simulink model "HinfModelLinear"  (R2018b)
settings: Solver=VariableStepAuto  StartTime=0.0  StopTime=20  RelTol=1e-3
undefined symbols (not defined in the file): A, B1, B2, C, K
libraries: cstblocks x1
settings Model: Creator=jban039  LastModifiedBy=jban039

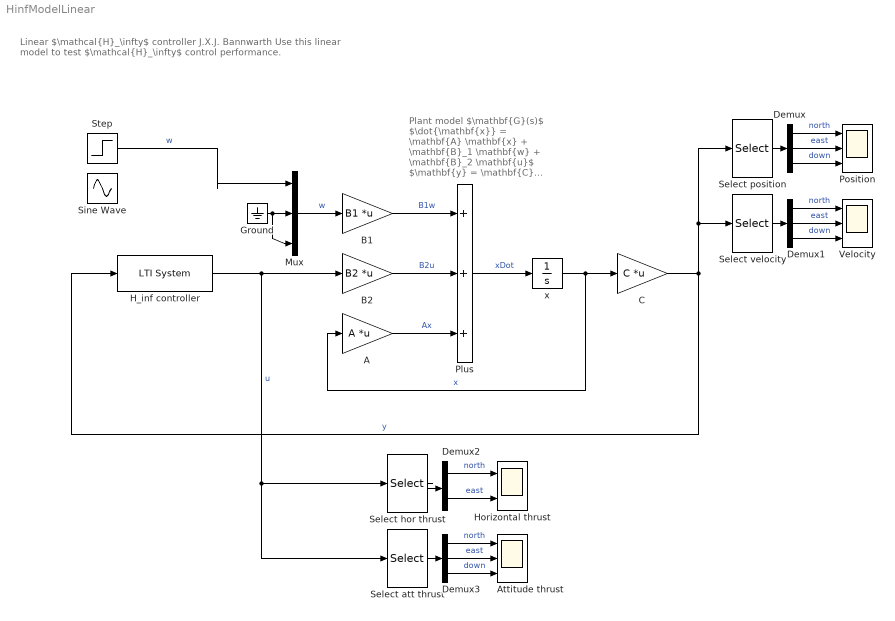
== system HinfModelLinear ==
  note: Linear $\mathcal{H}_\infty$ controller
      | J.X.J. Bannwarth
      |
      | Use this linear model to test $\mathcal{H}_\infty$ control performance.
  note: Plant model
      | $\mathbf{G}(s)$
      | $\dot{\mathbf{x}} = \mathbf{A} \mathbf{x} + \mathbf{B}_1 \mathbf{w} + \mathbf{B}_2 \mathbf{u}$
      | $\mathbf{y} = \mathbf{C} \mathbf{x}$
  A : Gain  Gain=A  Multiplication=Matrix(K*u)
  Attitude thrust : Scope  NumInputPorts=3
  B1 : Gain  Gain=B1  Multiplication=Matrix(K*u)
  B2 : Gain  Gain=B2  Multiplication=Matrix(K*u)
  C : Gain  Gain=C  Multiplication=Matrix(K*u)
  Demux : Demux  Outputs=3
  Demux1 : Demux  Outputs=3
  Demux2 : Demux  Outputs=2
  Demux3 : Demux  Outputs=3
  Ground : Ground
  H_inf controller : cstblocks/LTI System  sys=K  IC=[]
  Horizontal thrust : Scope  NumInputPorts=2
  Mux : Mux  Inputs=3
  Plus : Sum  Inputs=+++
  Position : Scope  NumInputPorts=3
  Select att thrust : Selector  InputPortWidth=size(K.D, 1)  IndexOptions=Index vector (dialog)  Indices=[3:5]  OutputSizes=1
  Select hor thrust : Selector  InputPortWidth=size(K.D, 1)  IndexOptions=Index vector (dialog)  Indices=[1:2]  OutputSizes=1
  Select position : Selector  InputPortWidth=size(C, 1)  IndexOptions=Index vector (dialog)  Indices=[4:6]  OutputSizes=1
  Select velocity : Selector  InputPortWidth=size(C, 1)  IndexOptions=Index vector (dialog)  Indices=[1:3]  OutputSizes=1
  Sine Wave : Sin  SampleTime=0
  Step : Step  After=5  SampleTime=0
  Velocity : Scope  NumInputPorts=3
  x : Integrator
  wires:
  x/1 -> C/1, A/1  "x"
  A/1 -> Plus/3  "Ax"
  Plus/1 -> x/1  "xDot"
  B1/1 -> Plus/1  "B1w"
  B2/1 -> Plus/2  "B2u"
  Mux/1 -> B1/1  "w"
  H_inf controller/1 -> Select att thrust/1, Select hor thrust/1, B2/1  "u"
  C/1 -> H_inf controller/1, Select velocity/1, Select position/1  "y"
  Demux/1 -> Position/1  "north"
  Demux/2 -> Position/2  "east"
  Demux/3 -> Position/3  "down"
  Select position/1 -> Demux/1
  Select velocity/1 -> Demux1/1
  Demux1/3 -> Velocity/3  "down"
  Demux1/2 -> Velocity/2  "east"
  Demux1/1 -> Velocity/1  "north"
  Step/1 -> Mux/1  "w"
  Ground/1 -> Mux/3, Mux/2
  Demux3/1 -> Attitude thrust/1  "north"
  Demux3/2 -> Attitude thrust/2  "east"
  Demux3/3 -> Attitude thrust/3  "down"
  Select att thrust/1 -> Demux3/1
  Select hor thrust/1 -> Demux2/1
  Demux2/2 -> Horizontal thrust/2  "east"
  Demux2/1 -> Horizontal thrust/1  "north"
